simulink model "sim_1dof"  (R2025b)
settings: Solver=ode45  StartTime=0.0  StopTime=Tend  MaxStep=1e-3*Ts  MinStep=1e-4*Ts  RelTol=1e-3
undefined symbols (not defined in the file): d1, d2, rho, Ts
libraries: cstblocks x2, simulink x1
settings Model: Creator=davidecovolo  LastModifiedBy=davidecovolo
settings SolverCC: InitialStep=1e-4*Ts

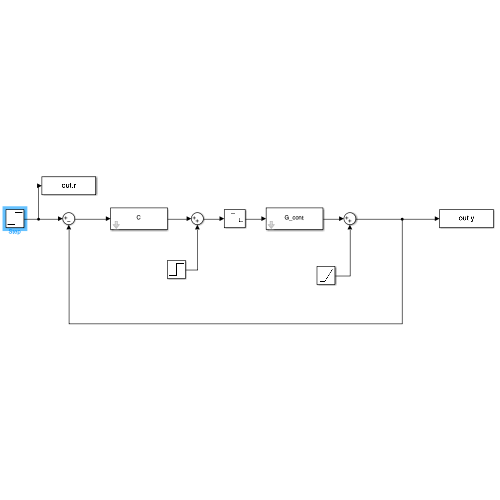
[thumbnail: Simulink's stored preview of the top-level diagram]
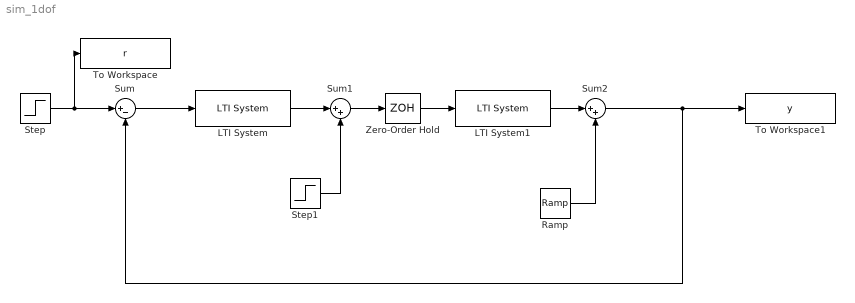
== system sim_1dof ==
  LTI System : cstblocks/LTI System  sys=C  IC=[]  PadeOrder=0
  LTI System1 : cstblocks/LTI System  sys=G_cont  IC=[]  PadeOrder=0
  Ramp : simulink/Sources/Ramp  slope=d2  start=0  InitialOutput=0
  Step : Step  Time=0  After=rho  SampleTime=Ts
  Step1 : Step  Time=0  After=d1  SampleTime=0
  Sum : Sum  Inputs=|+-
  Sum1 : Sum  Inputs=|++
  Sum2 : Sum  Inputs=|++
  To Workspace : ToWorkspace  VariableName=r  SaveFormat=Timeseries  SampleTime=Ts
  To Workspace1 : ToWorkspace  VariableName=y  SaveFormat=Timeseries  SampleTime=Ts
  Zero-Order Hold : ZeroOrderHold  SampleTime=Ts
  wires:
  LTI System/1 -> Sum1/1
  Zero-Order Hold/1 -> LTI System1/1
  Step/1 -> To Workspace/1, Sum/1
  Sum/1 -> LTI System/1
  Sum1/1 -> Zero-Order Hold/1
  Step1/1 -> Sum1/2
  LTI System1/1 -> Sum2/1
  Ramp/1 -> Sum2/2
  Sum2/1 -> Sum/2, To Workspace1/1
